simulink model "sampleModel1850"  (R2023a)
settings: Solver=VariableStepAuto  StartTime=0.0  StopTime=10.0  RelTol=1e-3
libraries: hdlsllib x7, simulink x3
settings Model: Creator=user1  LastModifiedBy=user1

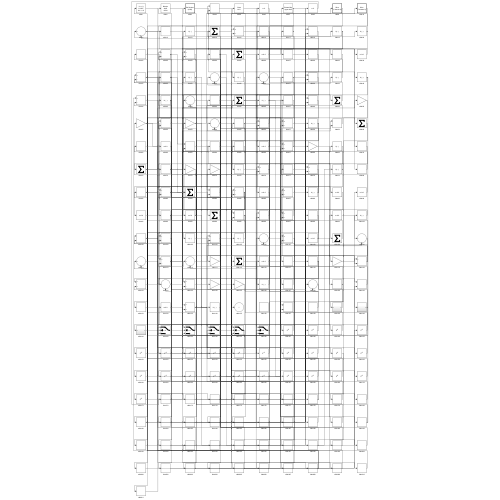
[thumbnail: Simulink's stored preview of the top-level diagram]
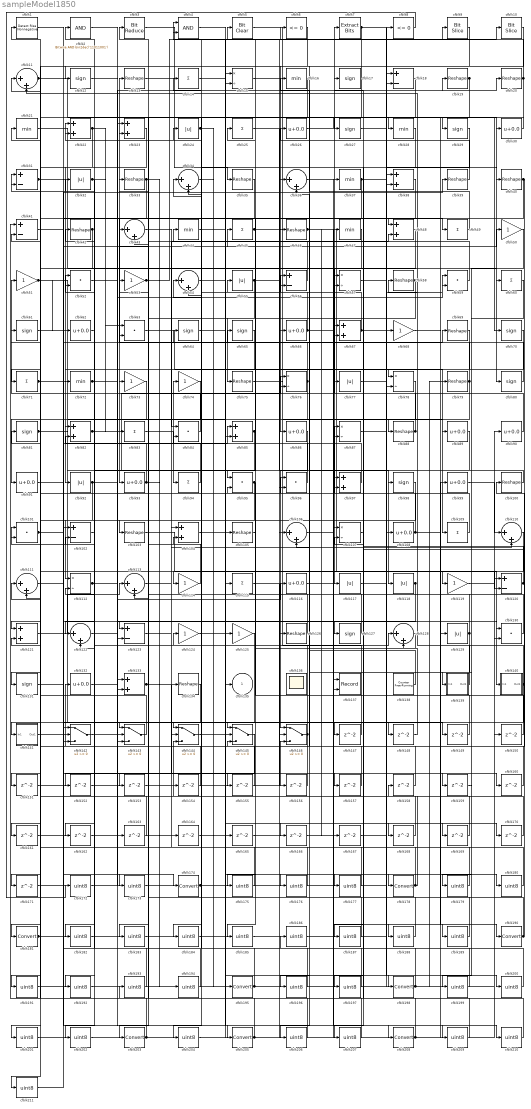
== system sampleModel1850 ==
  cfblk1 : hdlsllib/Logic and Bit Operations/Detect Rise Nonnegative  vinit=0  OutDataTypeStr=boolean
  cfblk10 : hdlsllib/Logic and Bit Operations/Bit Slice  lidx=7  ridx=0
  cfblk{13,19..20,33,35,39..40,42,46,58,69,75,79,88,100,103,105,126,134} (19 alike) : Reshape
  cfblk{52,59,63,84,95..96,101,130} (8 alike) : DotProduct  OutDataTypeStr=Inherit: Inherit via internal rule
  cfblk{18,31,41,56,102,120,123} (7 alike) : Sum  Inputs=+-
  cfblk{22..23,38,48,67,82,85,97,104,121,133} (11 alike) : Sum
  cfblk{11,34,36,43,54,106,110..111,113,122,128} (11 alike) : Sum  Inputs=|++
  cfblk{15,57,76,78,87,107,112} (7 alike) : Product  Inputs=*/  RndMeth=Zero  SaturateOnIntegerOverflow=on
  cfblk{26,30,62,66,86,89..91,93,99,108,116,132} (13 alike) : Bias  Bias=0.0  SaturateOnIntegerOverflow=off
  cfblk{14,25,45,49,60,71,83,94,109,115} (10 alike) : Sum  Inputs=+
  cfblk{50..51,53,68,73..74,114,119,124..125} (10 alike) : Gain
  cfblk{24,32,55,77,92,117..118,129} (8 alike) : Abs  SaturateOnIntegerOverflow=off
  cfblk{12,17,27,29,61,64..65,70,80..81,98,127,131} (13 alike) : Signum
  cfblk136 : Scope
      settings: Floating=on
  cfblk137 : Record  FileSettingsInternal="{\"entries\":[{\"content\":{\"excelSettings\":{\"content\":{},\"type\":\"Streamout.ExcelSettings\"}},\"type\":\"Streamout.FileSettingStorage\",\"uuid\":\"\"}],\"packageUris\":[\"http:\\/\\/schema.mathworks.com\\/mf0\\/streamout_blocks\\/R2020a\"],\"version\":\"1.0\"}"  Layout=[1 1]  SignalsInternal="{\"entries\":[{\"content\":{\"signals\":[{\"content\":{\"blockPath\":[],\"dimensions\":[1],\"domain\":\"\",\"lineColor\":\"#a2142f\",\"plots\":[1],\"port\":1,\"signalID\":4553,\"signalName\":\"XY Graph:1\"},\"type\":\"RecordBlkView.Signal\",\"uuid\":\"\"},{\"content\":{\"blockPath\":[],\"dimensions\":[1],\"domain\":\"\",\"lineColor\":\"#139fff\",\"plots\":[1],\"port\":2,\"signalID\":4556,\"signalName\":\"XY Graph:2\"},\"type\":\"RecordBlkView.Signal\",\"uuid\":\"\"}]},\"type\":\"RecordBlkView.InputSignals\",\"uuid\":\"\"}],\"packageUris\":[\"http:\\/\\/schema.mathworks.com\\/mf0\\/streamout_blocks\\/R2020a\"],\"version\":\"1.0\"}"  VisualizationBindings="{\"xyplotplugin\":{\"info\":[{\"series\":[{\"bindingParametersList\":[{\"parameter\":\"X-Axis\",\"signalID\":4553,\"signalName\":\"XY Graph:1\"},{\"parameter\":\"Y-Axis\",\"signalID\":4556,\"signalName\":\"XY Graph:2\"}],\"seriesID\":53753}],\"subplotID\":1}]}}"  CompatibilityTag=XY  st=-1
  cfblk138 : hdlsllib/Sources/Counter Free-Running  NumBits=16  tsamp=-1
  cfblk139 : Subsystem
      settings: LibrarySourceBlock=|
      | hdlsllib/Ports &
      | Subsystems/Subsystem
  cfblk140 : Subsystem
      settings: LibrarySourceBlock=|
      | hdlsllib/Ports &
      | Subsystems/Subsystem
  cfblk141 : Subsystem
      settings: LibrarySourceBlock=|
      | hdlsllib/Ports &
      | Subsystems/Subsystem
  cfblk{142..146} (5 alike) : Switch  SaturateOnIntegerOverflow=off  InputSameDT=off
  cfblk{147..171} (25 alike) : Delay  SampleTime=1
  cfblk{16,21,28,37,44,47,72} (7 alike) : MinMax
  cfblk{172..173,175..177,179..180,182..189,191..194,196..197,199..202,204,206..207,209..211} (31 alike) : DataTypeConversion  OutDataTypeStr=uint8  SaturateOnIntegerOverflow=off  RndMeth=Floor
  cfblk{174,178,181,190,195,198,203,205,208} (9 alike) : DataTypeConversion  SaturateOnIntegerOverflow=off  RndMeth=Floor
  cfblk2 : simulink/Logic and Bit Operations/Bitwise Operator  logicop=AND  UseBitMask=on  BitMask=bin2dec('11011001')  BitMaskRealWorld=Stored Integer
      settings: LibrarySourceBlock=|
      | hdlsllib/Logic and Bit
      | Operations/Bitwise
      | Operator
  cfblk3 : hdlsllib/Logic and Bit Operations/Bit Reduce  mode=AND
  cfblk4 : Logic  AllPortsSameDT=off  OutDataTypeStr=boolean
  cfblk5 : simulink/Logic and Bit Operations/Bit Clear  iBit=0
      settings: LibrarySourceBlock=|
      | hdlsllib/Logic and Bit
      | Operations/Bit Clear
  cfblk6 : hdlsllib/Logic and Bit Operations/Compare To Zero  relop=<=  OutDataTypeStr=boolean
  cfblk7 : simulink/Logic and Bit Operations/Extract Bits  bitsToExtract=Upper half  numBits=8  bitIdxRange=[0 7]  outScalingMode=Preserve fixed-point scaling
      settings: LibrarySourceBlock=|
      | hdlsllib/Logic and Bit
      | Operations/Extract Bits
  cfblk8 : hdlsllib/Logic and Bit Operations/Compare To Zero  relop=<=  OutDataTypeStr=boolean
  cfblk9 : hdlsllib/Logic and Bit Operations/Bit Slice  lidx=7  ridx=0
  cfblk135 : Outport  VectorParamsAs1DForOutWhenUnconnected=off
  wires:
  cfblk140/1(Out1) -> cfblk11/2, cfblk185/1
  cfblk118/1 -> cfblk127/1, cfblk133/2
  cfblk53/1 -> cfblk10/1, cfblk134/1
  cfblk88/1 -> cfblk7/1, cfblk77/1
  cfblk15/1 -> cfblk128/1
  cfblk33/1 -> cfblk93/1, cfblk194/1
  cfblk81/1 -> cfblk145/1, cfblk153/1
  cfblk40/1 -> cfblk132/1, cfblk71/1
  cfblk20/1 -> cfblk80/1, cfblk4/2
  cfblk85/1 -> cfblk31/1, cfblk122/1, cfblk122/2
  cfblk42/1 -> cfblk92/1, cfblk121/1
  cfblk128/1 -> cfblk55/1
  cfblk51/1 -> cfblk118/1, cfblk62/1
  cfblk142/1 -> cfblk208/1
  cfblk22/1 -> cfblk82/1, cfblk83/1
  cfblk68/1 -> cfblk190/1
  cfblk121/1 -> cfblk113/1
  cfblk127/1 -> cfblk5/1
  cfblk78/1 -> cfblk88/1
  cfblk76/1 -> cfblk13/1, cfblk171/1
  cfblk13/1 -> cfblk35/1
  cfblk86/1 -> cfblk146/1
  cfblk29/1 -> cfblk114/1
  cfblk45/1 -> cfblk78/1, cfblk97/1
  cfblk103/1 -> cfblk119/1
  cfblk114/1 -> cfblk33/1
  cfblk101/1 -> cfblk64/1, cfblk173/1
  cfblk19/1 -> cfblk144/1, cfblk143/2
  cfblk139/1(Out1) -> cfblk58/1
  cfblk83/1 -> cfblk94/1
  cfblk119/1 -> cfblk90/1
  cfblk9/1 -> cfblk86/1
  cfblk96/1 -> cfblk74/1
  cfblk133/1 -> cfblk48/2, cfblk159/1, cfblk160/1
  cfblk37/1 -> cfblk95/1, cfblk169/1
  cfblk49/1 -> cfblk26/1
  cfblk99/1 -> cfblk110/1
  cfblk71/1 -> cfblk115/1, cfblk50/1
  cfblk97/1 -> cfblk52/1
  cfblk63/1 -> cfblk109/1
  cfblk58/1 -> cfblk75/1, cfblk103/1
  cfblk35/1 -> cfblk73/1
  cfblk21/1 -> cfblk117/1
  cfblk46/1 -> cfblk140/1(In1), cfblk167/1
  cfblk72/1 -> cfblk133/1, cfblk20/1
  cfblk23/1 -> cfblk131/1
  cfblk130/1 -> cfblk56/1
  cfblk131/1 -> cfblk39/1
  cfblk74/1 -> cfblk113/2
  cfblk92/1 -> cfblk69/1, cfblk211/1
  cfblk3/1 -> cfblk30/1
  cfblk32/1 -> cfblk63/1, cfblk182/1
  cfblk108/1 -> cfblk87/1, cfblk120/2
  cfblk43/1 -> cfblk84/1
  cfblk73/1 -> cfblk91/1
  cfblk105/1 -> cfblk65/1
  cfblk80/1 -> cfblk24/1
  cfblk7/1 -> cfblk49/1, cfblk46/1
  cfblk61/1 -> cfblk174/1
  cfblk129/1 -> cfblk36/2, cfblk196/1
  cfblk55/1 -> cfblk9/1, cfblk145/2
  cfblk109/1 -> cfblk81/1
  cfblk67/1 -> cfblk22/1, cfblk59/1
  cfblk48/1 -> cfblk66/1
  cfblk66/1 -> cfblk14/1, cfblk189/1
  cfblk54/1 -> cfblk198/1
  cfblk75/1 -> cfblk89/1
  cfblk120/1 -> cfblk17/1, cfblk97/2
  cfblk11/1 -> cfblk70/1, cfblk48/1
  cfblk25/1 -> cfblk60/1
  cfblk70/1 -> cfblk72/1
  cfblk18/1 -> cfblk181/1
  cfblk31/1 -> cfblk67/1, cfblk143/3
  cfblk90/1 -> cfblk51/1
  cfblk146/1 -> cfblk101/1, cfblk145/3
  cfblk91/1 -> cfblk85/1
  cfblk60/1 -> cfblk139/1(In1)
  cfblk82/1 -> cfblk135/1, cfblk15/2, cfblk147/1
  cfblk113/1 -> cfblk110/2
  cfblk84/1 -> cfblk2/1
  cfblk10/1 -> cfblk106/2
  cfblk95/1 -> cfblk112/1, cfblk175/1
  cfblk100/1 -> cfblk98/1
  cfblk5/1 -> cfblk129/1
  cfblk12/1 -> cfblk130/1
  cfblk93/1 -> cfblk3/1, cfblk52/2, cfblk164/1
  cfblk41/1 -> cfblk205/1
  cfblk126/1 -> cfblk53/1
  cfblk2/1 -> cfblk27/1
  cfblk1/1 -> cfblk123/1
  cfblk34/1 -> cfblk195/1
  cfblk79/1 -> cfblk141/1(In1), cfblk25/1
  cfblk123/1 -> cfblk76/1
  cfblk104/1 -> cfblk178/1
  cfblk17/1 -> cfblk12/1, cfblk126/1
  cfblk87/1 -> cfblk19/1
  cfblk39/1 -> cfblk16/1
  cfblk138/1 -> cfblk96/1
  cfblk26/1 -> cfblk29/1
  cfblk94/1 -> cfblk42/1
  cfblk30/1 -> cfblk28/1
  cfblk98/1 -> cfblk111/2
  cfblk122/1 -> cfblk116/1
  cfblk56/1 -> cfblk23/2
  cfblk59/1 -> cfblk4/1
  cfblk116/1 -> cfblk137/1
  cfblk24/1 -> cfblk165/1, cfblk204/1
  cfblk112/1 -> cfblk45/1, cfblk59/2, cfblk202/1
  cfblk65/1 -> cfblk143/1
  cfblk14/1 -> cfblk6/1
  cfblk125/1 -> cfblk203/1
  cfblk27/1 -> cfblk40/1
  cfblk143/1 -> cfblk11/1
  cfblk147/1 -> cfblk22/2
  cfblk106/1 -> cfblk148/1
  cfblk148/1 -> cfblk128/2
  cfblk141/1(Out1) -> cfblk149/1
  cfblk149/1 -> cfblk57/1
  cfblk150/1 -> cfblk95/2
  cfblk110/1 -> cfblk151/1
  cfblk151/1 -> cfblk144/3
  cfblk145/1 -> cfblk152/1
  cfblk152/1 -> cfblk15/1
  cfblk153/1 -> cfblk146/3
  cfblk154/1 -> cfblk23/1
  cfblk132/1 -> cfblk155/1
  cfblk155/1 -> cfblk82/2
  cfblk115/1 -> cfblk156/1
  cfblk156/1 -> cfblk31/2
  cfblk111/1 -> cfblk157/1
  cfblk157/1 -> cfblk56/2
  cfblk158/1 -> cfblk84/2
  cfblk160/1 -> cfblk112/2
  cfblk6/1 -> cfblk161/1
  cfblk161/1 -> cfblk67/2
  cfblk62/1 -> cfblk162/1
  cfblk162/1 -> cfblk85/2
  cfblk52/1 -> cfblk163/1
  cfblk163/1 -> cfblk1/1
  cfblk164/1 -> cfblk76/2
  cfblk165/1 -> cfblk87/2
  cfblk4/1 -> cfblk166/1
  cfblk167/1 -> cfblk78/2
  cfblk124/1 -> cfblk168/1
  cfblk168/1 -> cfblk146/2
  cfblk169/1 -> cfblk101/2
  cfblk117/1 -> cfblk170/1
  cfblk170/1 -> cfblk144/2
  cfblk171/1 -> cfblk123/2
  cfblk8/1 -> cfblk172/1
  cfblk172/1 -> cfblk108/1
  cfblk173/1 -> cfblk8/1
  cfblk174/1 -> cfblk105/1, cfblk124/1
  cfblk175/1 -> cfblk61/1
  cfblk44/1 -> cfblk176/1
  cfblk176/1 -> cfblk32/1
  cfblk64/1 -> cfblk177/1
  cfblk177/1 -> cfblk44/1
  cfblk178/1 -> cfblk158/1, cfblk111/1
  cfblk50/1 -> cfblk179/1
  cfblk179/1 -> cfblk104/1
  cfblk77/1 -> cfblk180/1
  cfblk180/1 -> cfblk104/2
  cfblk181/1 -> cfblk96/2, cfblk57/2
  cfblk182/1 -> cfblk18/1
  cfblk16/1 -> cfblk183/1
  cfblk183/1 -> cfblk18/2
  cfblk38/1 -> cfblk184/1
  cfblk184/1 -> cfblk106/1
  cfblk185/1 -> cfblk38/1
  cfblk186/1 -> cfblk38/2
  cfblk107/1 -> cfblk187/1
  cfblk187/1 -> cfblk43/1
  cfblk36/1 -> cfblk188/1
  cfblk188/1 -> cfblk107/1
  cfblk189/1 -> cfblk107/2
  cfblk190/1 -> cfblk43/2, cfblk100/1
  cfblk134/1 -> cfblk191/1
  cfblk191/1 -> cfblk68/1
  cfblk102/1 -> cfblk192/1
  cfblk192/1 -> cfblk130/2
  cfblk193/1 -> cfblk102/1
  cfblk194/1 -> cfblk102/2
  cfblk195/1 -> cfblk154/1, cfblk137/2
  cfblk196/1 -> cfblk34/1
  cfblk69/1 -> cfblk197/1
  cfblk197/1 -> cfblk34/2
  cfblk198/1 -> cfblk186/1, cfblk79/1
  cfblk159/1 -> cfblk199/1
  cfblk199/1 -> cfblk54/1
  cfblk57/1 -> cfblk200/1
  cfblk200/1 -> cfblk54/2
  cfblk47/1 -> cfblk201/1
  cfblk201/1 -> cfblk120/1
  cfblk202/1 -> cfblk47/1
  cfblk203/1 -> cfblk193/1, cfblk36/1
  cfblk204/1 -> cfblk125/1
  cfblk205/1 -> cfblk150/1, cfblk63/2, cfblk99/1
  cfblk89/1 -> cfblk206/1
  cfblk206/1 -> cfblk41/1
  cfblk28/1 -> cfblk207/1
  cfblk207/1 -> cfblk41/2
  cfblk208/1 -> cfblk121/2, cfblk21/1, cfblk37/1
  cfblk166/1 -> cfblk209/1
  cfblk209/1 -> cfblk142/1
  cfblk144/1 -> cfblk210/1
  cfblk210/1 -> cfblk142/2
  cfblk211/1 -> cfblk142/3

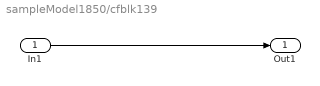
== system sampleModel1850/cfblk139 ==
  In1 : Inport
  Out1 : Outport
  wires:
  In1/1 -> Out1/1

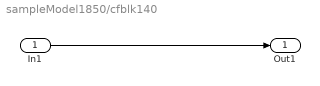
== system sampleModel1850/cfblk140 ==
  In1 : Inport
  Out1 : Outport
  wires:
  In1/1 -> Out1/1

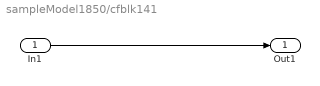
== system sampleModel1850/cfblk141 ==
  In1 : Inport
  Out1 : Outport
  wires:
  In1/1 -> Out1/1
